simulink model "validate_observer"  (R2015a)
settings: Solver=FixedStepDiscrete  StartTime=0.0  StopTime=T  FixedStep=0.02  RelTol=1e-3
values from neighbouring files (symbols this model uses):
  A = stateModelMatrices(1:l-1, 1:l-1)    [controller_design_1.m]    (also in controller_design_2.m)
  B = stateModelMatrices(1:l-1, l)    [controller_design_1.m]    (also in controller_design_2.m)
  C = stateModelMatrices(l, 1:l-1)    [controller_design_1.m]    (also in controller_design_2.m)
  D = stateModelMatrices(l, l)    [controller_design_1.m]    (also in controller_design_2.m)
undefined symbols (not defined in the file or in its folder): M
settings Model: Creator=alunos  LastModifiedBy=luisr
settings DataIOCC: LimitDataPoints=off

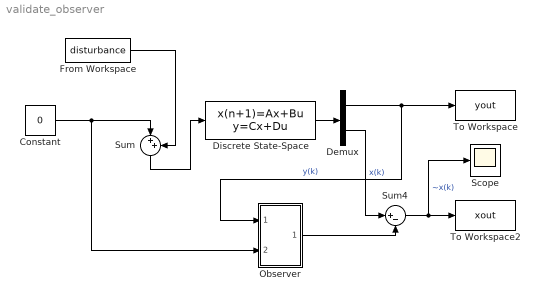
== system validate_observer ==
  Constant : Constant  Value=0
  Demux : Demux  Outputs=[1 4]
  Discrete State-Space : DiscreteStateSpace  A=A  B=B  C=[C; eye(length(A))]  D=[D; zeros(size(A,1),1)]  SampleTime=0.02
  From Workspace : FromWorkspace  VariableName=disturbance  SampleTime=[0.02,0]
  Observer : Subsystem
  Scope : Scope
      settings: TimeRange=auto  MaxDataPoints=5000  SaveToWorkspace=off  SaveName=ScopeData  YMin=-1.32807  YMax=1.32791  SampleTime=-1
  Sum : Sum  Inputs=|++
  Sum4 : Sum  Inputs=|+-
  To Workspace : ToWorkspace  VariableName=yout  SaveFormat=Structure With Time  SampleTime=-1
  To Workspace2 : ToWorkspace  VariableName=xout  SaveFormat=Structure With Time  SampleTime=-1
  wires:
  Discrete State-Space/1 -> Demux/1
  Demux/1 -> Observer/1(In1), To Workspace/1  "y(k)"
  From Workspace/1 -> Sum/2
  Sum/1 -> Discrete State-Space/1
  Constant/1 -> Observer/2(In2), Sum/1
  Sum4/1 -> Scope/1, To Workspace2/1  "~x(k)"
  Demux/2 -> Sum4/1  "x(k)"
  Observer/1(Out1) -> Sum4/2

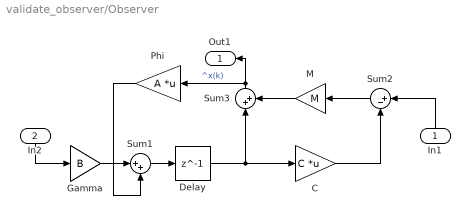
== system validate_observer/Observer ==
  In1 : Inport
  In2 : Inport  Port=2
  C : Gain  Gain=C  Multiplication=Matrix(K*u)
  Delay : Delay  DelayLength=1  InitialCondition=0  SampleTime=[0.02,0]
  Gamma : Gain  Gain=B
  M : Gain  Gain=M
  Phi : Gain  Gain=A  Multiplication=Matrix(K*u)
  Sum1 : Sum  Inputs=|++
  Sum2 : Sum  Inputs=|+-
  Sum3 : Sum  Inputs=|++
  Out1 : Outport
  wires:
  Gamma/1 -> Sum1/1
  Sum3/1 -> Out1/1, Phi/1  "^x(k)"
  Phi/1 -> Sum1/2
  Sum1/1 -> Delay/1
  M/1 -> Sum3/2
  C/1 -> Sum2/2
  Delay/1 -> Sum3/1, C/1
  Sum2/1 -> M/1
  In2/1 -> Gamma/1
  In1/1 -> Sum2/1
